simulink model "bldc_sim"  (R2024b)
settings: Solver=VariableStepAuto  StartTime=0.0  StopTime=3  RelTol=1e-3
values from neighbouring files (symbols this model uses):
  D_m = 0.001    [setup_motor_params.m]
  J = 0.1    [setup_motor_params.m]
  Ke = 0.1    [setup_motor_params.m]
  Kt = P/2 * lambda_m    (= 0.2)    [setup_motor_params.m]
  L_ss = 0.002    [setup_motor_params.m]
  lambda_m = 0.1    [setup_motor_params.m]
  P = 4    [setup_motor_params.m]
  phi_A_deg = 9.0 * 0    (= 0)    [setup_motor_params.m]
  phi_B_deg = -1.0 * 0    (= 0)    [setup_motor_params.m]
  phi_C_deg = 7.0* 0    (= 0)    [setup_motor_params.m]
  R_s = 0.7    [setup_motor_params.m]
  tau_s = L_ss/R_s    (= 0.00285714285714)    [setup_motor_params.m]
  Ts_motor = 1e-6    (= 1e-06)    [setup_motor_params.m]
libraries: ee_lib x9, nesl_utility x9, embmathops x2, fl_lib x2, spsPWMGeneratorDCDCLib x1
(part 1 of 2)
settings Model: Creator=Aether  LastModifiedBy=Aether

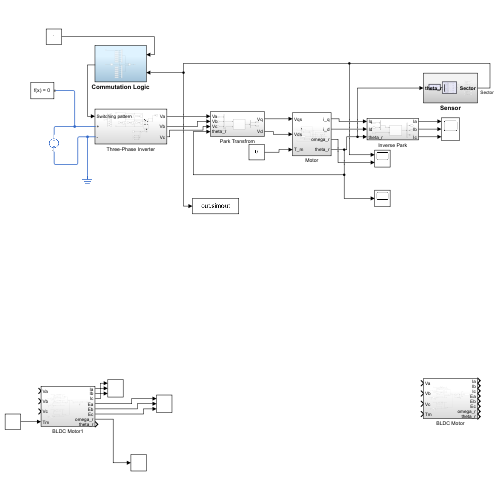
[thumbnail: Simulink's stored preview of the top-level diagram]
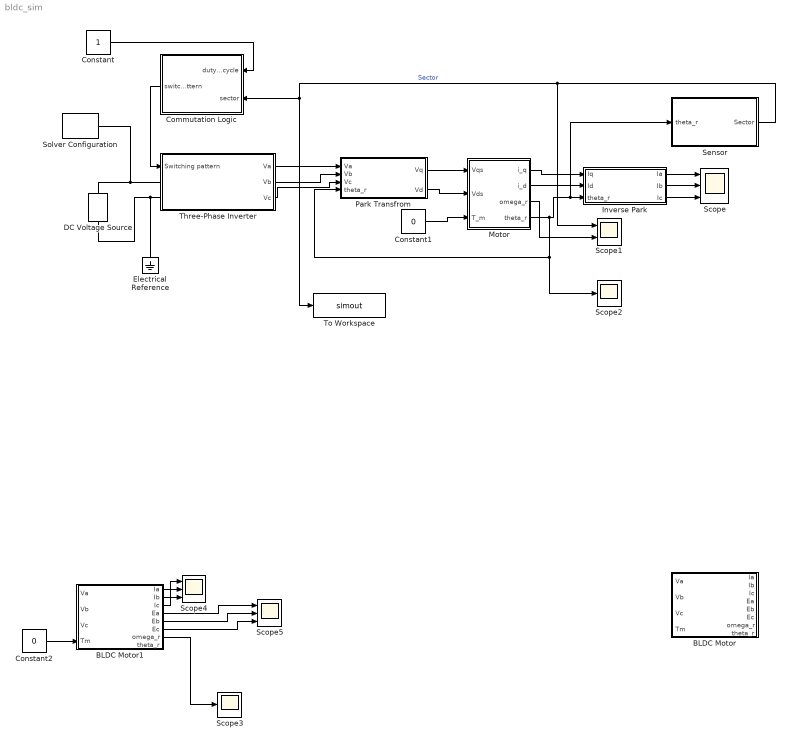
== system bldc_sim ==
  BLDC Motor : Subsystem
  BLDC Motor1 : Subsystem
  Commutation Logic : Subsystem
  Constant : Constant
  Constant1 : Constant  Value=0
  Constant2 : Constant  Value=0
  DC Voltage Source : ee_lib/Additional Components/SPICE Sources/DC Voltage Source  DC=36 V
  Electrical Reference : fl_lib/Electrical/Electrical Elements/Electrical Reference
  Inverse Park : Subsystem
  Motor : Subsystem
  Park Transfrom : Subsystem
  Scope : Scope  NumInputPorts=3
  Scope1 : Scope  NumInputPorts=2
  Scope2 : Scope
  Scope3 : Scope
  Scope4 : Scope  NumInputPorts=3
  Scope5 : Scope  NumInputPorts=3
  Sensor : Subsystem
  Solver Configuration : nesl_utility/Solver Configuration  PhysicalDomain=network_engine_domain  SubClassName=solver  LeftPortType=input  RightPortType=generic  Tones=[]  Harmonics=[]  SimulateNoise=off  Profile=off  UseLocalSampling=off  EnableSwitchedLinearOptims=on  FrequencyDomain=off  UseCCode=off  RelTol=0.001  AbsTol=0.001  MinStep=1e-09  ToWorkspace=off  RevertToSquareIcSolve=off  NumHomotopyIterations=100  PhasorMode=off  PhasorModeNumHarmonics=1  ConsistencySolver=NEWTON_XTOL_AFTER_FTOL  IndexReductionMethod=DerivativeReplacement  DoDC=off  ResidualTolerance=1e-09  ConsistencyTolSource=GLOBAL  ConsistencyAbsTol=0.001  ConsistencyRelTol=0.001  ConsistencyTolFactor=0.001  UseLocalSolver=off  LocalSolverChoice=NE_BACKWARD_EULER_ADVANCER  ResolveIndetEquations=on  FunctionEvalNumThread=1  LocalSolverSampleTime=0.001  DoFixedCost=off  MaxNonlinIter=3  MaxModeIter=2  ComputeImpulses=off  ImpulseIterations=2  LinearAlgebra=auto  LinearAlgebraNumThread=0  EquationFormulation=NE_TIME_EF  DelaysMemoryBudget=1024  AutomaticFiltering=on  FilteringTimeConstant=0.001  PartitionStorageMethod=AS_NEEDED  PartitionMemoryBudget=1024  PartitionMethod=ROBUST  MultibodyUseLocalSolver=off  MultibodyLocalSolverChoice=ODE1  MultibodyLocalSolverSampleTime=0.001
  Three-Phase Inverter : Subsystem
  To Workspace : ToWorkspace  VariableName=simout  SaveFormat=Timeseries  SampleTime=-1
  wires:
  Constant/1 -> Commutation Logic/1(duty_cycle)
  Commutation Logic/1("  switching_pattern") -> Three-Phase Inverter/1(Switching pattern)
  Park Transfrom/1(Vq) -> Motor/1(Vqs)
  Park Transfrom/2(Vd) -> Motor/2(Vds)
  Motor/1(i_q) -> Inverse Park/1(Iq)
  Motor/2(i_d) -> Inverse Park/2(Id)
  Motor/4(theta_r) -> Scope2/1, Park Transfrom/4(theta_r), Sensor/1(theta_r), Inverse Park/3(theta_r)
  Inverse Park/1(Ia) -> Scope/1
  Inverse Park/2(Ib) -> Scope/2
  Inverse Park/3(Ic) -> Scope/3
  Sensor/1(Sector) -> Scope1/1, Commutation Logic/2(sector), To Workspace/1  "Sector"
  Constant1/1 -> Motor/3(T_m)
  Motor/3(omega_r) -> Scope1/2
  Constant2/1 -> BLDC Motor1/4(Tm)
  BLDC Motor1/1(Ia) -> Scope4/1
  BLDC Motor1/2(Ib) -> Scope4/2
  BLDC Motor1/3(Ic) -> Scope4/3
  BLDC Motor1/7(omega_r) -> Scope3/1
  BLDC Motor1/4(Ea) -> Scope5/1
  BLDC Motor1/5(Eb) -> Scope5/2
  BLDC Motor1/6(Ec) -> Scope5/3
  Three-Phase Inverter/1(Va) -> Park Transfrom/1(Va)
  Three-Phase Inverter/2(Vb) -> Park Transfrom/2(Vb)
  Three-Phase Inverter/3(Vc) -> Park Transfrom/3(Vc)
  connections:
  DC Voltage Source/LConn1 -- Solver Configuration/RConn1 -- Three-Phase Inverter/LConn1
  DC Voltage Source/RConn1 -- Electrical Reference/LConn1 -- Three-Phase Inverter/LConn2

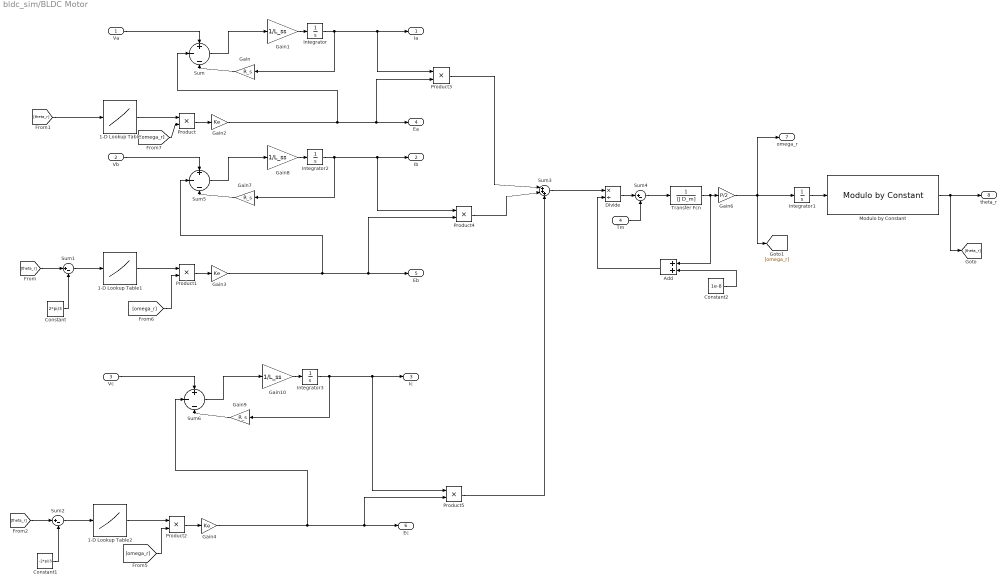
== system bldc_sim/BLDC Motor ==
  Va : Inport
  Vb : Inport  Port=2
  Vc : Inport  Port=3
  Tm : Inport  Port=4
  1-D Lookup Table : Lookup_n-D  NumberOfTableDimensions=1  BreakpointsForDimension1=[0, pi/3, 2*pi/3, pi, 4*pi/3, 5*pi/3, 2*pi]  Table=[0, 1, 1, 0, -1, -1, 0]  InternalRulePriority=Speed  RndMeth=Simplest
  1-D Lookup Table1 : Lookup_n-D  NumberOfTableDimensions=1  BreakpointsForDimension1=[0, pi/3, 2*pi/3, pi, 4*pi/3, 5*pi/3, 2*pi]  Table=[0, 1, 1, 0, -1, -1, 0]  InternalRulePriority=Speed  RndMeth=Simplest
  1-D Lookup Table2 : Lookup_n-D  NumberOfTableDimensions=1  BreakpointsForDimension1=[0, pi/3, 2*pi/3, pi, 4*pi/3, 5*pi/3, 2*pi]  Table=[0, 1, 1, 0, -1, -1, 0]  InternalRulePriority=Speed  RndMeth=Simplest
  Add : Sum
  Constant : Constant  Value=2*pi/3
  Constant1 : Constant  Value=-2*pi/3
  Constant2 : Constant  Value=1e-8
  Divide : Product  Inputs=*/
  Gain : Gain  Gain=R_s
  Gain1 : Gain  Gain=1/L_ss
  Gain10 : Gain  Gain=1/L_ss
  Gain2 : Gain  Gain=Ke
  Gain3 : Gain  Gain=Ke
  Gain4 : Gain  Gain=Ke
  Gain6 : Gain  Gain=P/2
  Gain7 : Gain  Gain=R_s
  Gain8 : Gain  Gain=1/L_ss
  Gain9 : Gain  Gain=R_s
  Integrator : Integrator
  Integrator1 : Integrator  InitialCondition=0.1
  Integrator2 : Integrator
  Integrator3 : Integrator
  Modulo by Constant : embmathops/Modulo by Constant  Denominator=2*pi  SimulateUsing=Code generation
      settings: LibrarySourceBlock=embeddedMathLib/Modulo by Constant
  Product{,1..5} (6 alike) : Product
  Sum : Sum  Inputs=+|-|-
  Sum1 : Sum  Inputs=|+-
  Sum2 : Sum  Inputs=|+-
  Sum3 : Sum  Inputs=|+++
  Sum4 : Sum  Inputs=|+-
  Sum5 : Sum  Inputs=+|-|-
  Sum6 : Sum  Inputs=+|-|-
  Transfer Fcn : TransferFcn  Denominator=[J D_m]
  Ia : Outport
  Ib : Outport  Port=2
  Ic : Outport  Port=3
  Ea : Outport  Port=4
  Eb : Outport  Port=5
  Ec : Outport  Port=6
  omega_r : Outport  Port=7
  theta_r : Outport  Port=8
  wires:
  Va/1 -> Sum/1
  Gain/1 -> Sum/3
  Sum/1 -> Gain1/1
  Gain1/1 -> Integrator/1
  Integrator/1 -> Product3/1, Ia/1, Gain/1
  1-D Lookup Table/1 -> Product/1
  Product/1 -> Gain2/1
  Gain2/1 -> Sum/2, Product3/2, Ea/1
  Product1/1 -> Gain3/1
  1-D Lookup Table1/1 -> Product1/1
  Gain3/1 -> Sum5/2, Product4/2, Eb/1
  Sum1/1 -> 1-D Lookup Table1/1
  Constant/1 -> Sum1/2
  Gain4/1 -> Sum6/2, Product5/2, Ec/1
  Constant1/1 -> Sum2/2
  1-D Lookup Table2/1 -> Product2/1
  Product2/1 -> Gain4/1
  Sum2/1 -> 1-D Lookup Table2/1
  Product3/1 -> Sum3/1
  Product4/1 -> Sum3/2
  Product5/1 -> Sum3/3
  Sum3/1 -> Divide/1
  Divide/1 -> Sum4/1
  Tm/1 -> Sum4/2
  Sum4/1 -> Transfer Fcn/1
  Transfer Fcn/1 -> Add/1, Gain6/1
  Gain6/1 -> omega_r/1, [omega_r], Integrator1/1
  Integrator1/1 -> Modulo by Constant/1
  Gain7/1 -> Sum5/3
  Gain8/1 -> Integrator2/1
  Sum5/1 -> Gain8/1
  Vb/1 -> Sum5/1
  Integrator2/1 -> Product4/1, Ib/1, Gain7/1
  Vc/1 -> Sum6/1
  Gain9/1 -> Sum6/3
  Gain10/1 -> Integrator3/1
  Integrator3/1 -> Product5/1, Ic/1, Gain9/1
  Sum6/1 -> Gain10/1
  Modulo by Constant/1 -> [theta_r], theta_r/1
  [theta_r] -> Sum1/1
  [theta_r] -> Sum2/1
  [omega_r] -> Product2/2
  [omega_r] -> Product1/2
  [omega_r] -> Product/2
  [theta_r] -> 1-D Lookup Table/1
  Constant2/1 -> Add/2
  Add/1 -> Divide/2

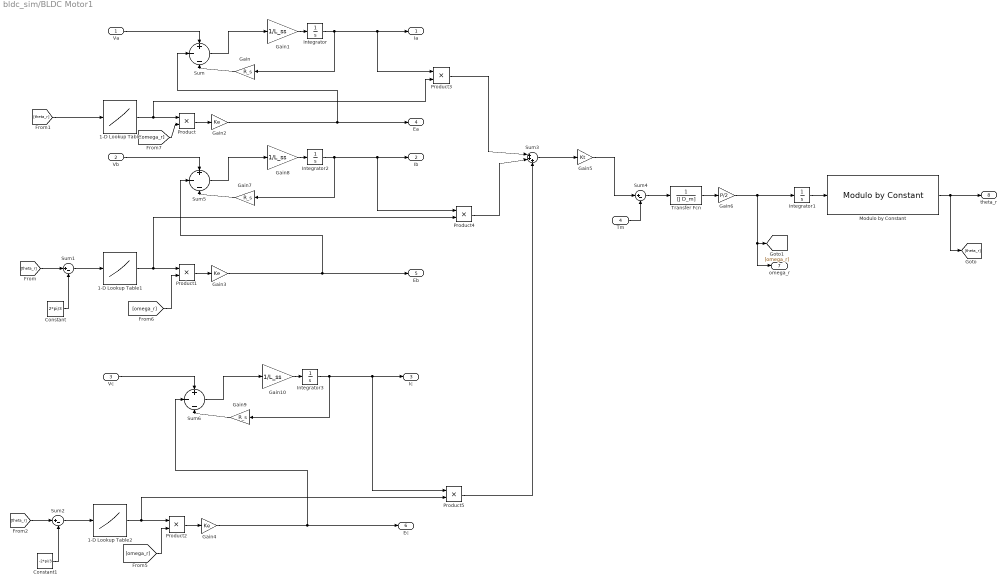
== system bldc_sim/BLDC Motor1 ==
  Va : Inport
  Vb : Inport  Port=2
  Vc : Inport  Port=3
  Tm : Inport  Port=4
  1-D Lookup Table : Lookup_n-D  NumberOfTableDimensions=1  BreakpointsForDimension1=[0, pi/3, 2*pi/3, pi, 4*pi/3, 5*pi/3, 2*pi]  Table=[0, 1, 1, 0, -1, -1, 0]  InternalRulePriority=Speed  RndMeth=Simplest
  1-D Lookup Table1 : Lookup_n-D  NumberOfTableDimensions=1  BreakpointsForDimension1=[0, pi/3, 2*pi/3, pi, 4*pi/3, 5*pi/3, 2*pi]  Table=[0, 1, 1, 0, -1, -1, 0]  InternalRulePriority=Speed  RndMeth=Simplest
  1-D Lookup Table2 : Lookup_n-D  NumberOfTableDimensions=1  BreakpointsForDimension1=[0, pi/3, 2*pi/3, pi, 4*pi/3, 5*pi/3, 2*pi]  Table=[0, 1, 1, 0, -1, -1, 0]  InternalRulePriority=Speed  RndMeth=Simplest
  Constant : Constant  Value=2*pi/3
  Constant1 : Constant  Value=-2*pi/3
  Gain : Gain  Gain=R_s
  Gain1 : Gain  Gain=1/L_ss
  Gain10 : Gain  Gain=1/L_ss
  Gain2 : Gain  Gain=Ke
  Gain3 : Gain  Gain=Ke
  Gain4 : Gain  Gain=Ke
  Gain5 : Gain  Gain=Kt
  Gain6 : Gain  Gain=P/2
  Gain7 : Gain  Gain=R_s
  Gain8 : Gain  Gain=1/L_ss
  Gain9 : Gain  Gain=R_s
  Integrator : Integrator
  Integrator1 : Integrator  InitialCondition=0.1
  Integrator2 : Integrator
  Integrator3 : Integrator
  Modulo by Constant : embmathops/Modulo by Constant  Denominator=2*pi  SimulateUsing=Code generation
  Product{,1..5} (6 alike) : Product
  Sum : Sum  Inputs=+|-|-
  Sum1 : Sum  Inputs=|+-
  Sum2 : Sum  Inputs=|+-
  Sum3 : Sum  Inputs=|+++
  Sum4 : Sum  Inputs=|+-
  Sum5 : Sum  Inputs=+|-|-
  Sum6 : Sum  Inputs=+|-|-
  Transfer Fcn : TransferFcn  Denominator=[J D_m]
  Ia : Outport
  Ib : Outport  Port=2
  Ic : Outport  Port=3
  Ea : Outport  Port=4
  Eb : Outport  Port=5
  Ec : Outport  Port=6
  omega_r : Outport  Port=7
  theta_r : Outport  Port=8
  wires:
  Va/1 -> Sum/1
  Gain/1 -> Sum/3
  Sum/1 -> Gain1/1
  Gain1/1 -> Integrator/1
  Integrator/1 -> Product3/1, Ia/1, Gain/1
  1-D Lookup Table/1 -> Product3/2, Product/1
  Product/1 -> Gain2/1
  Gain2/1 -> Sum/2, Ea/1
  Product1/1 -> Gain3/1
  1-D Lookup Table1/1 -> Product4/2, Product1/1
  Gain3/1 -> Sum5/2, Eb/1
  Sum1/1 -> 1-D Lookup Table1/1
  Constant/1 -> Sum1/2
  Gain4/1 -> Sum6/2, Ec/1
  Constant1/1 -> Sum2/2
  1-D Lookup Table2/1 -> Product5/2, Product2/1
  Product2/1 -> Gain4/1
  Sum2/1 -> 1-D Lookup Table2/1
  Gain5/1 -> Sum4/1
  Tm/1 -> Sum4/2
  Sum4/1 -> Transfer Fcn/1
  Transfer Fcn/1 -> Gain6/1
  Gain6/1 -> omega_r/1, [omega_r], Integrator1/1
  Integrator1/1 -> Modulo by Constant/1
  Gain7/1 -> Sum5/3
  Gain8/1 -> Integrator2/1
  Sum5/1 -> Gain8/1
  Vb/1 -> Sum5/1
  Integrator2/1 -> Product4/1, Ib/1, Gain7/1
  Vc/1 -> Sum6/1
  Gain9/1 -> Sum6/3
  Gain10/1 -> Integrator3/1
  Integrator3/1 -> Product5/1, Ic/1, Gain9/1
  Sum6/1 -> Gain10/1
  Modulo by Constant/1 -> [theta_r], theta_r/1
  [theta_r] -> Sum1/1
  [theta_r] -> Sum2/1
  [omega_r] -> Product2/2
  [omega_r] -> Product1/2
  [omega_r] -> Product/2
  [theta_r] -> 1-D Lookup Table/1
  Product3/1 -> Sum3/1
  Product4/1 -> Sum3/2
  Product5/1 -> Sum3/3
  Sum3/1 -> Gain5/1

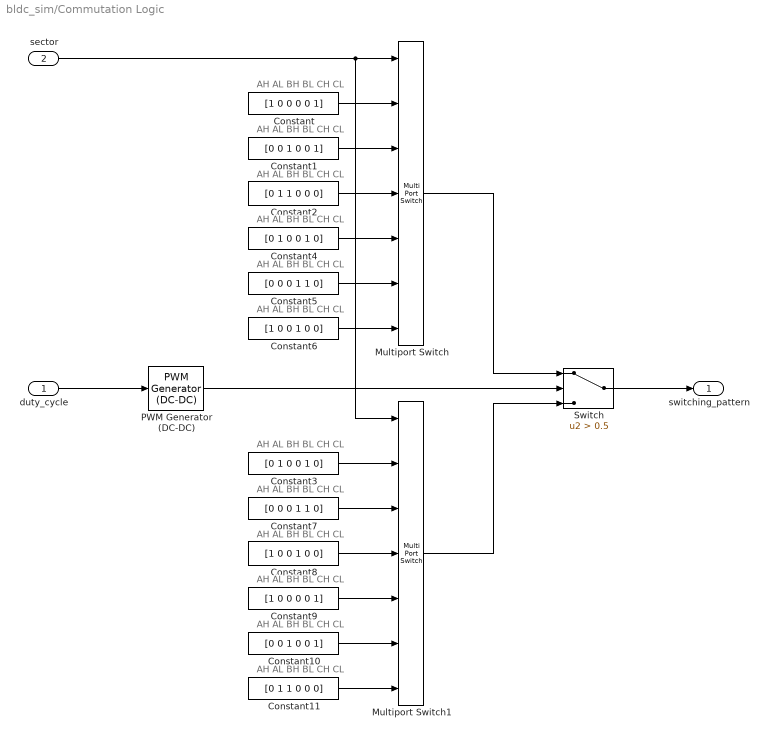
== system bldc_sim/Commutation Logic ==
  note: AH AL BH BL CH CL
  note: AH AL BH BL CH CL
  note: AH AL BH BL CH CL
  note: AH AL BH BL CH CL
  note: AH AL BH BL CH CL
  note: AH AL BH BL CH CL
  note: AH AL BH BL CH CL
  note: AH AL BH BL CH CL
  note: AH AL BH BL CH CL
  note: AH AL BH BL CH CL
  note: AH AL BH BL CH CL
  note: AH AL BH BL CH CL
  duty_cycle : Inport
  sector : Inport  Port=2
  Constant : Constant  Value=[1 0 0 0 0 1]
  Constant1 : Constant  Value=[0 0 1 0 0 1]
  Constant10 : Constant  Value=[0 0 1 0 0 1]
  Constant11 : Constant  Value=[0 1 1 0 0 0]
  Constant2 : Constant  Value=[0 1 1 0 0 0]
  Constant3 : Constant  Value=[0 1 0 0 1 0]
  Constant4 : Constant  Value=[0 1 0 0 1 0]
  Constant5 : Constant  Value=[0 0 0 1 1 0]
  Constant6 : Constant  Value=[1 0 0 1 0 0]
  Constant7 : Constant  Value=[0 0 0 1 1 0]
  Constant8 : Constant  Value=[1 0 0 1 0 0]
  Constant9 : Constant  Value=[1 0 0 0 0 1]
  Multiport Switch : MultiPortSwitch  Inputs=6  SaturateOnIntegerOverflow=off  InputSameDT=off
  Multiport Switch1 : MultiPortSwitch  Inputs=6  SaturateOnIntegerOverflow=off  InputSameDT=off
  PWM Generator (DC-DC) : spsPWMGeneratorDCDCLib/PWM Generator (DC-DC)  Fsw=1e7  Ts=Ts_motor
  Switch : Switch  Criteria=u2 > Threshold  Threshold=0.5  SaturateOnIntegerOverflow=off  InputSameDT=off
  "  switching_pattern" : Outport  VectorParamsAs1DForOutWhenUnconnected=off
  wires:
  Constant6/1 -> Multiport Switch/7
  Constant4/1 -> Multiport Switch/5
  sector/1 -> Multiport Switch1/1, Multiport Switch/1
  Constant1/1 -> Multiport Switch/3
  Constant2/1 -> Multiport Switch/4
  Constant5/1 -> Multiport Switch/6
  Constant/1 -> Multiport Switch/2
  Constant9/1 -> Multiport Switch1/5
  Constant11/1 -> Multiport Switch1/7
  Constant3/1 -> Multiport Switch1/2
  Constant7/1 -> Multiport Switch1/3
  Constant10/1 -> Multiport Switch1/6
  Constant8/1 -> Multiport Switch1/4
  PWM Generator (DC-DC)/1 -> Switch/2
  Switch/1 -> "  switching_pattern"/1
  Multiport Switch/1 -> Switch/1
  Multiport Switch1/1 -> Switch/3
  duty_cycle/1 -> PWM Generator (DC-DC)/1

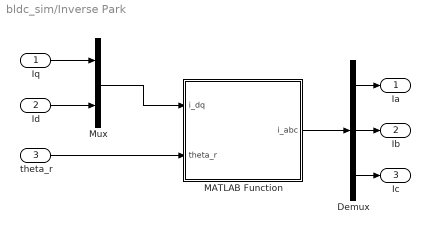
== system bldc_sim/Inverse Park ==
  Iq : Inport
  Id : Inport  Port=2
  theta_r : Inport  Port=3
  Demux : Demux  Outputs=3
  MATLAB Function : MATLAB Function  TreatAsAtomicUnit=on
  Mux : Mux  Inputs=2
  Ia : Outport
  Ib : Outport  Port=2
  Ic : Outport  Port=3
  wires:
  Mux/1 -> MATLAB Function/1(i_dq)
  theta_r/1 -> MATLAB Function/2(theta_r)
  MATLAB Function/1(i_abc) -> Demux/1
  Id/1 -> Mux/2
  Iq/1 -> Mux/1
  Demux/1 -> Ia/1
  Demux/2 -> Ib/1
  Demux/3 -> Ic/1

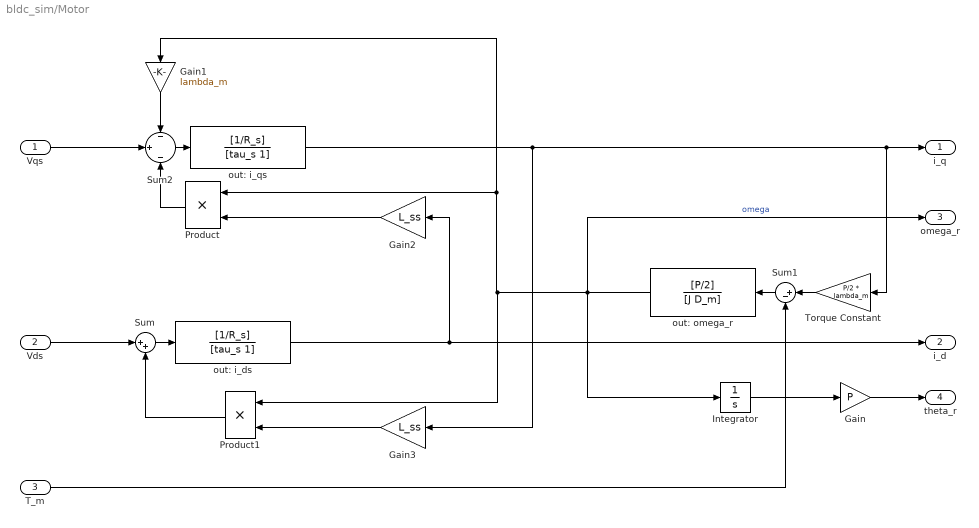
== system bldc_sim/Motor ==
  Vqs : Inport
  Vds : Inport  Port=2
  T_m : Inport  Port=3
  Gain : Gain  Gain=P
  Gain1 : Gain  Gain=lambda_m
  Gain2 : Gain  Gain=L_ss
  Gain3 : Gain  Gain=L_ss
  Integrator : Integrator
  Product : Product
  Product1 : Product
  Sum : Sum  Inputs=|++
  Sum1 : Sum  Inputs=|+-
  Sum2 : Sum  Inputs=-|+|-
  Torque Constant : Gain  Gain=P/2 * lambda_m
  out: i_ds : TransferFcn  Numerator=[1/R_s]  Denominator=[tau_s 1]
  out: i_qs : TransferFcn  Numerator=[1/R_s]  Denominator=[tau_s 1]
  out: omega_r : TransferFcn  Numerator=[P/2]  Denominator=[J D_m]
  i_q : Outport
  i_d : Outport  Port=2
  omega_r : Outport  Port=3
  theta_r : Outport  Port=4
  wires:
  Sum2/1 -> out: i_qs/1
  Gain2/1 -> Product/2
  Vqs/1 -> Sum2/2
  out: i_qs/1 -> i_q/1, Torque Constant/1, Gain3/1
  out: omega_r/1 -> omega_r/1, Integrator/1, Product1/1, Product/1, Gain1/1  "omega"
  Gain1/1 -> Sum2/1
  out: i_ds/1 -> i_d/1, Gain2/1
  Integrator/1 -> Gain/1
  T_m/1 -> Sum1/2
  Sum1/1 -> out: omega_r/1
  Sum/1 -> out: i_ds/1
  Torque Constant/1 -> Sum1/1
  Product/1 -> Sum2/3
  Gain3/1 -> Product1/2
  Vds/1 -> Sum/1
  Product1/1 -> Sum/2
  Gain/1 -> theta_r/1

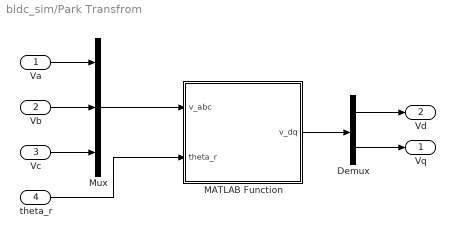
== system bldc_sim/Park Transfrom ==
  Va : Inport
  Vb : Inport  Port=2
  Vc : Inport  Port=3
  theta_r : Inport  Port=4
  Demux : Demux  Outputs=2
  MATLAB Function : MATLAB Function  TreatAsAtomicUnit=on
  Mux : Mux  Inputs=3
  Vq : Outport
  Vd : Outport  Port=2
  wires:
  theta_r/1 -> MATLAB Function/2(theta_r)
  Vb/1 -> Mux/2
  Va/1 -> Mux/1
  Vc/1 -> Mux/3
  Mux/1 -> MATLAB Function/1(v_abc)
  MATLAB Function/1(v_dq) -> Demux/1
  Demux/1 -> Vd/1
  Demux/2 -> Vq/1

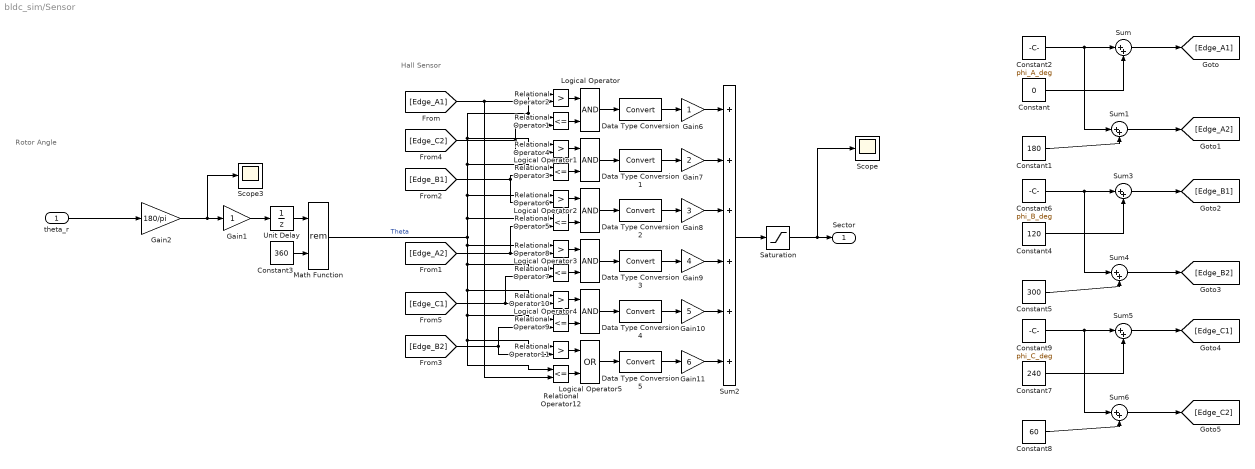
== system bldc_sim/Sensor ==
  note: Rotor Angle
  note: Hall Sensor
  theta_r : Inport
  Constant : Constant  Value=0
  Constant1 : Constant  Value=180
  Constant2 : Constant  Value=phi_A_deg
  Constant3 : Constant  Value=360
  Constant4 : Constant  Value=120
  Constant5 : Constant  Value=300
  Constant6 : Constant  Value=phi_B_deg
  Constant7 : Constant  Value=240
  Constant8 : Constant  Value=60
  Constant9 : Constant  Value=phi_C_deg
  Data Type Conversion{,1..5} (6 alike) : DataTypeConversion
  Gain1 : Gain
  Gain10 : Gain  Gain=5  SaturateOnIntegerOverflow=on  OutDataTypeStr=Inherit: Same as input  ParamDataTypeStr=Inherit: Same as input
  Gain11 : Gain  Gain=6  SaturateOnIntegerOverflow=on  OutDataTypeStr=Inherit: Same as input  ParamDataTypeStr=Inherit: Same as input
  Gain2 : Gain  Gain=180/pi
  Gain6 : Gain  SaturateOnIntegerOverflow=on  OutDataTypeStr=Inherit: Same as input  ParamDataTypeStr=Inherit: Same as input
  Gain7 : Gain  Gain=2  SaturateOnIntegerOverflow=on  OutDataTypeStr=Inherit: Same as input  ParamDataTypeStr=Inherit: Same as input
  Gain8 : Gain  Gain=3  SaturateOnIntegerOverflow=on  OutDataTypeStr=Inherit: Same as input  ParamDataTypeStr=Inherit: Same as input
  Gain9 : Gain  Gain=4  SaturateOnIntegerOverflow=on  OutDataTypeStr=Inherit: Same as input  ParamDataTypeStr=Inherit: Same as input
  Logical Operator{,1..4} (5 alike) : Logic
  Logical Operator5 : Logic  Operator=OR
  Math Function : Math  Operator=rem  SignedPower=on
  Relational Operator{1,3,5,7,9,12} (6 alike) : RelationalOperator  Operator=<=
  Relational Operator{2,4,6,8,10..11} (6 alike) : RelationalOperator  Operator=>
  Saturation : Saturate  UpperLimit=6  LowerLimit=1
  Scope : Scope
  Scope3 : Scope
  Sum{,1,3..6} (6 alike) : Sum  Inputs=|++
  Sum2 : Sum  Inputs=++++++  InputSameDT=on  SaturateOnIntegerOverflow=on  OutDataTypeStr=Inherit: Same as first input
  Unit Delay : UnitDelay  SampleTime=Ts_motor  HasFrameUpgradeWarning=on
  Sector : Outport
  wires:
  Saturation/1 -> Scope/1, Sector/1
  Math Function/1 -> Relational Operator2/1, Relational Operator1/1, Relational Operator4/1, Relational Operator3/1, Relational Operator6/1, Relational Operator5/1, Relational Operator12/1, Relational Operator11/1, Relational Operator9/1, Relational Operator10/1, Relational Operator7/1, Relational Operator8/1  "Theta"
  Data Type Conversion5/1 -> Gain11/1
  Data Type Conversion4/1 -> Gain10/1
  Data Type Conversion3/1 -> Gain9/1
  Data Type Conversion2/1 -> Gain8/1
  Data Type Conversion1/1 -> Gain7/1
  Data Type Conversion/1 -> Gain6/1
  Relational Operator2/1 -> Logical Operator/1
  Relational Operator1/1 -> Logical Operator/2
  Logical Operator/1 -> Data Type Conversion/1
  [Edge_A1] -> Relational Operator12/2, Relational Operator2/2
  Relational Operator4/1 -> Logical Operator1/1
  Relational Operator3/1 -> Logical Operator1/2
  Logical Operator1/1 -> Data Type Conversion1/1
  [Edge_C2] -> Relational Operator1/2, Relational Operator4/2
  Relational Operator6/1 -> Logical Operator2/1
  Relational Operator5/1 -> Logical Operator2/2
  Logical Operator2/1 -> Data Type Conversion2/1
  Relational Operator8/1 -> Logical Operator3/1
  Relational Operator7/1 -> Logical Operator3/2
  Logical Operator3/1 -> Data Type Conversion3/1
  Relational Operator10/1 -> Logical Operator4/1
  Relational Operator9/1 -> Logical Operator4/2
  Logical Operator4/1 -> Data Type Conversion4/1
  Relational Operator11/1 -> Logical Operator5/1
  Relational Operator12/1 -> Logical Operator5/2
  Logical Operator5/1 -> Data Type Conversion5/1
  Gain6/1 -> Sum2/1
  Gain7/1 -> Sum2/2
  Gain8/1 -> Sum2/3
  Gain9/1 -> Sum2/4
  Gain10/1 -> Sum2/5
  Gain11/1 -> Sum2/6
  Sum2/1 -> Saturation/1
  Gain2/1 -> Scope3/1, Gain1/1
  Constant3/1 -> Math Function/2
  Gain1/1 -> Unit Delay/1
  Unit Delay/1 -> Math Function/1
  Constant/1 -> Sum/2
  Constant2/1 -> Sum1/1, Sum/1
  Constant1/1 -> Sum1/2
  Sum/1 -> [Edge_A1]
  Sum1/1 -> [Edge_A2]
  Constant6/1 -> Sum4/1, Sum3/1
  Constant5/1 -> Sum4/2
  Constant4/1 -> Sum3/2
  Sum3/1 -> [Edge_B1]
  Sum4/1 -> [Edge_B2]
  Constant9/1 -> Sum6/1, Sum5/1
  Constant8/1 -> Sum6/2
  Constant7/1 -> Sum5/2
  Sum5/1 -> [Edge_C1]
  Sum6/1 -> [Edge_C2]
  [Edge_B1] -> Relational Operator3/2, Relational Operator6/2
  [Edge_A2] -> Relational Operator5/2, Relational Operator8/2
  [Edge_C1] -> Relational Operator7/2, Relational Operator10/2
  [Edge_B2] -> Relational Operator11/2, Relational Operator9/2
  theta_r/1 -> Gain2/1
